simulink model "a1_climbing"  (R2022b)
settings: Solver=VariableStepAuto  StartTime=0.0  StopTime=5  RelTol=1e-3
values from neighbouring files (symbols this model uses):
  m = 12    [MPC_Controller.m]    (also in QP_Controller.m; TASK1_rotating_mpc.m; TASK1_walking_backward_mpc.m; TASK1_walking_forward_mpc.m)
  N = 10    [MPC_Controller.m]
undefined symbols (not defined in the file or in its folder): climbing_mpc, X, Y, Z
libraries: sm_lib x206, nesl_utility x122, simulink x1
(part 6 of 6)

== system a1_climbing/Stand Controller/Subsystem9 ==
  angle : Inport
  velocity : Inport  Port=2
  Add : Sum
  Constant1 : Constant  Value=-0.5
  Constant2 : Constant  Value=-5
  Constant3 : Constant  Value=0
  Product : Product
  Product1 : Product
  Saturation : Saturate  UpperLimit=33.5  LowerLimit=-33.5
  Subtract : Sum  Inputs=+-
  Torque : Outport
  wires:
  angle/1 -> Subtract/1
  Constant2/1 -> Product/2
  Subtract/1 -> Product/1
  Constant1/1 -> Product1/2
  velocity/1 -> Product1/1
  Product1/1 -> Add/2
  Product/1 -> Add/1
  Constant3/1 -> Subtract/2
  Add/1 -> Saturation/1
  Saturation/1 -> Torque/1

== system a1_climbing/Walk Controller/Convert Forces to Torque1 ==
  F : Inport
  RR_Ang_Vec : Inport  Port=2
  RL_Ang_Vec : Inport  Port=3
  FL_Ang_Vec : Inport  Port=4
  FR_Ang_Vec : Inport  Port=5
  Force to Torque : MATLAB Function  TreatAsAtomicUnit=on
  Tau_FL : Outport
  Tau_RL : Outport  Port=2
  Tau_FR : Outport  Port=3
  Tau_RR : Outport  Port=4
  wires:
  F/1 -> Force to Torque/1(F)
  Force to Torque/1(Tau_RR) -> Tau_RR/1
  Force to Torque/2(Tau_FR) -> Tau_FR/1
  Force to Torque/3(Tau_FL) -> Tau_FL/1
  Force to Torque/4(Tau_RL) -> Tau_RL/1
  RR_Ang_Vec/1 -> Force to Torque/2(RR_ang_vec)
  RL_Ang_Vec/1 -> Force to Torque/3(RL_ang_vec)
  FL_Ang_Vec/1 -> Force to Torque/4(FL_ang_vec)
  FR_Ang_Vec/1 -> Force to Torque/5(FR_ang_vec)

== system a1_climbing/Walk Controller/Rigid Body Controller ==
  FL Pos : Inport
  RL Pos : Inport  Port=2
  FR Pos : Inport  Port=3
  RR Pos : Inport  Port=4
  COM_pos : Inport  Port=5
  COM_vel : Inport  Port=6
  COM_ang_vel : Inport  Port=7
  Rot : Inport  Port=8
  v_desired : Inport  Port=9
  T_stance : Inport  Port=10
  Clock : Clock
  Interpreted MATLAB Function : MATLABFcn  MATLABFcn=climbing_mpc(u)  OutputDimensions=12  Output1D=off
  Memory : Memory
  Mux : Mux  Inputs=11
  Rotation Matrix to Eul : MATLAB Function  TreatAsAtomicUnit=on
  Scope : Scope  NumInputPorts=5
  Selector : Selector  InputPortWidth=12  IndexOptions=Index vector (dialog)  Indices=[1 3]  OutputSizes=1
  Zero-Order Hold : ZeroOrderHold  SampleTime=.05
  u : Outport
  wires:
  COM_pos/1 -> Mux/1
  COM_vel/1 -> Mux/2
  COM_ang_vel/1 -> Mux/4
  FL Pos/1 -> Mux/5
  RL Pos/1 -> Mux/6
  FR Pos/1 -> Mux/7
  RR Pos/1 -> Mux/8
  Rot/1 -> Rotation Matrix to Eul/1(u)
  Rotation Matrix to Eul/1(y) -> Mux/3
  Interpreted MATLAB Function/1 -> Memory/1
  Memory/1 -> Selector/1, u/1
  Mux/1 -> Zero-Order Hold/1
  Zero-Order Hold/1 -> Interpreted MATLAB Function/1
  Clock/1 -> Mux/9
  Selector/1 -> Scope/1
  v_desired/1 -> Mux/10
  T_stance/1 -> Mux/11

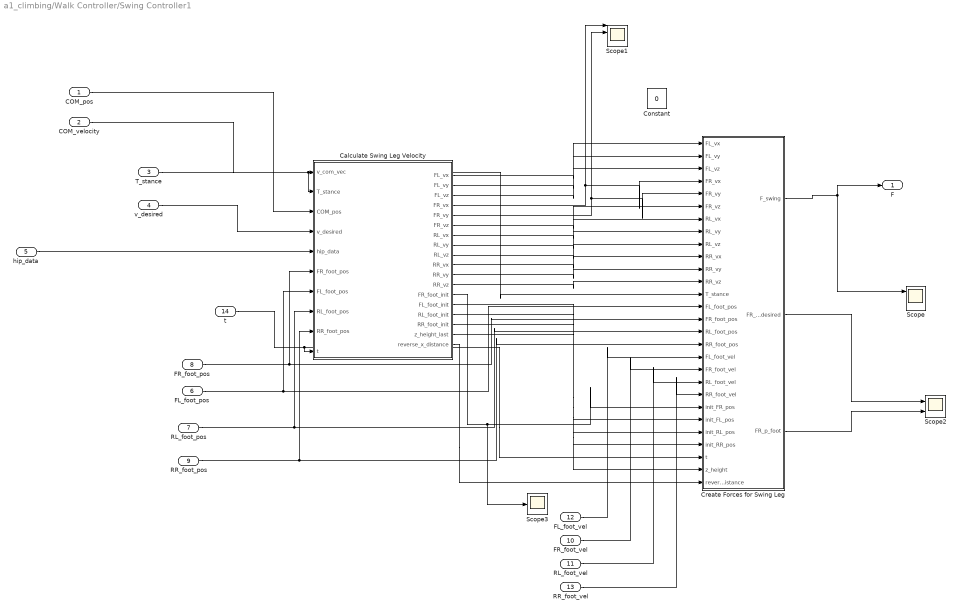
== system a1_climbing/Walk Controller/Swing Controller1 ==
  COM_pos : Inport
  COM_velocity : Inport  Port=2
  T_stance : Inport  Port=3
  v_desired : Inport  Port=4
  hip_data : Inport  Port=5
  FL_foot_pos : Inport  Port=6
  RL_foot_pos : Inport  Port=7
  FR_foot_pos : Inport  Port=8
  RR_foot_pos : Inport  Port=9
  FR_foot_vel : Inport  Port=10
  RL_foot_vel : Inport  Port=11
  FL_foot_vel : Inport  Port=12
  RR_foot_vel : Inport  Port=13
  t : Inport  Port=14
  Calculate Swing Leg Velocity : MATLAB Function  TreatAsAtomicUnit=on  SystemSampleTime=0.2
  Constant : Constant  Value=0
  Create Forces for Swing Leg : MATLAB Function  TreatAsAtomicUnit=on
  Scope : Scope  NumInputPorts=3
  Scope1 : Scope  NumInputPorts=4
  Scope2 : Scope  NumInputPorts=2
  Scope3 : Scope
  F : Outport
  wires:
  T_stance/1 -> Calculate Swing Leg Velocity/2(T_stance), Create Forces for Swing Leg/13(T_stance)
  v_desired/1 -> Calculate Swing Leg Velocity/4(v_desired)
  Create Forces for Swing Leg/1(F_swing) -> Scope/1, F/1
  t/1 -> Calculate Swing Leg Velocity/10(t), Create Forces for Swing Leg/26(t)
  hip_data/1 -> Calculate Swing Leg Velocity/5(hip_data)
  Calculate Swing Leg Velocity/12(RR_vz) -> Create Forces for Swing Leg/12(RR_vz)
  Calculate Swing Leg Velocity/11(RR_vy) -> Create Forces for Swing Leg/11(RR_vy)
  Calculate Swing Leg Velocity/10(RR_vx) -> Create Forces for Swing Leg/10(RR_vx)
  Calculate Swing Leg Velocity/9(RL_vz) -> Create Forces for Swing Leg/9(RL_vz)
  Calculate Swing Leg Velocity/8(RL_vy) -> Create Forces for Swing Leg/8(RL_vy)
  Calculate Swing Leg Velocity/7(RL_vx) -> Create Forces for Swing Leg/7(RL_vx)
  Calculate Swing Leg Velocity/6(FR_vz) -> Create Forces for Swing Leg/6(FR_vz)
  Calculate Swing Leg Velocity/5(FR_vy) -> Create Forces for Swing Leg/5(FR_vy), Scope1/2
  Calculate Swing Leg Velocity/4(FR_vx) -> Create Forces for Swing Leg/4(FR_vx), Scope1/1
  Calculate Swing Leg Velocity/3(FL_vz) -> Create Forces for Swing Leg/3(FL_vz)
  Calculate Swing Leg Velocity/2(FL_vy) -> Create Forces for Swing Leg/2(FL_vy)
  Calculate Swing Leg Velocity/1(FL_vx) -> Create Forces for Swing Leg/1(FL_vx)
  FR_foot_pos/1 -> Create Forces for Swing Leg/15(FR_foot_pos), Calculate Swing Leg Velocity/6(FR_foot_pos)
  RL_foot_pos/1 -> Calculate Swing Leg Velocity/8(RL_foot_pos), Create Forces for Swing Leg/16(RL_foot_pos)
  RR_foot_pos/1 -> Create Forces for Swing Leg/17(RR_foot_pos), Calculate Swing Leg Velocity/9(RR_foot_pos)
  FL_foot_vel/1 -> Create Forces for Swing Leg/18(FL_foot_vel)
  FR_foot_vel/1 -> Create Forces for Swing Leg/19(FR_foot_vel)
  RL_foot_vel/1 -> Create Forces for Swing Leg/20(RL_foot_vel)
  RR_foot_vel/1 -> Create Forces for Swing Leg/21(RR_foot_vel)
  Create Forces for Swing Leg/2(FR_p_desired) -> Scope2/1
  COM_velocity/1 -> Calculate Swing Leg Velocity/1(v_com_vec)
  Calculate Swing Leg Velocity/13(FR_foot_init) -> Scope3/1, Create Forces for Swing Leg/22(init_FR_pos)
  Create Forces for Swing Leg/3(FR_p_foot) -> Scope2/2
  FL_foot_pos/1 -> Calculate Swing Leg Velocity/7(FL_foot_pos), Create Forces for Swing Leg/14(FL_foot_pos)
  Calculate Swing Leg Velocity/14(FL_foot_init) -> Create Forces for Swing Leg/23(init_FL_pos)
  Calculate Swing Leg Velocity/15(RL_foot_init) -> Create Forces for Swing Leg/24(init_RL_pos)
  Calculate Swing Leg Velocity/16(RR_foot_init) -> Create Forces for Swing Leg/25(init_RR_pos)
  COM_pos/1 -> Calculate Swing Leg Velocity/3(COM_pos)
  Calculate Swing Leg Velocity/17(z_height_last) -> Create Forces for Swing Leg/27(z_height)
  Calculate Swing Leg Velocity/18(reverse_x_distance) -> Create Forces for Swing Leg/28(reverse_x_distance)

== matlab function a1_climbing/Rear Right Leg/Separate Torques ==
  data: torque_vector input; hip_torque output; thigh_torque output; calf_torque output
function [hip_torque, thigh_torque, calf_torque] = fcn(torque_vector)

hip_torque = torque_vector(1);
thigh_torque = torque_vector(2);
calf_torque = torque_vector(3);

== matlab function a1_climbing/Front Left Leg/Separate Torques ==
  data: torque_vector input; hip_torque output; thigh_torque output; calf_torque output
function [hip_torque, thigh_torque, calf_torque] = fcn(torque_vector)

hip_torque = torque_vector(1);
thigh_torque = torque_vector(2);
calf_torque = torque_vector(3);

== matlab function a1_climbing/Stand Controller/MATLAB Function ==
  data: angle_vector input; hip_angle output; thigh_angle output; calf_angle output
function [hip_angle, thigh_angle, calf_angle] = fcn(angle_vector)

hip_angle = angle_vector(1);
thigh_angle = angle_vector(2);
calf_angle = angle_vector(3);

== matlab function a1_climbing/Stand Controller/MATLAB Function1 ==
  data: velocity_vector input; hip_velocity output; thigh_velocity output; calf_velocity output
function [hip_velocity, thigh_velocity, calf_velocity] = fcn(velocity_vector)

hip_velocity = velocity_vector(1);
thigh_velocity = velocity_vector(2);
calf_velocity = velocity_vector(3);

== matlab function a1_climbing/Stand Controller/MATLAB Function2 ==
  data: angle_vector input; hip_angle output; thigh_angle output; calf_angle output
function [hip_angle, thigh_angle, calf_angle] = fcn(angle_vector)

hip_angle = angle_vector(1);
thigh_angle = angle_vector(2);
calf_angle = angle_vector(3);

== matlab function a1_climbing/Stand Controller/MATLAB Function3 ==
  data: velocity_vector input; hip_velocity output; thigh_velocity output; calf_velocity output
function [hip_velocity, thigh_velocity, calf_velocity] = fcn(velocity_vector)

hip_velocity = velocity_vector(1);
thigh_velocity = velocity_vector(2);
calf_velocity = velocity_vector(3);

== matlab function a1_climbing/Stand Controller/MATLAB Function4 ==
  data: angle_vector input; hip_angle output; thigh_angle output; calf_angle output
function [hip_angle, thigh_angle, calf_angle] = fcn(angle_vector)

hip_angle = angle_vector(1);
thigh_angle = angle_vector(2);
calf_angle = angle_vector(3);

== matlab function a1_climbing/Stand Controller/MATLAB Function5 ==
  data: velocity_vector input; hip_velocity output; thigh_velocity output; calf_velocity output
function [hip_velocity, thigh_velocity, calf_velocity] = fcn(velocity_vector)

hip_velocity = velocity_vector(1);
thigh_velocity = velocity_vector(2);
calf_velocity = velocity_vector(3);

== matlab function a1_climbing/Stand Controller/MATLAB Function6 ==
  data: angle_vector input; hip_angle output; thigh_angle output; calf_angle output
function [hip_angle, thigh_angle, calf_angle] = fcn(angle_vector)

hip_angle = angle_vector(1);
thigh_angle = angle_vector(2);
calf_angle = angle_vector(3);

== matlab function a1_climbing/Stand Controller/MATLAB Function7 ==
  data: velocity_vector input; hip_velocity output; thigh_velocity output; calf_velocity output
function [hip_velocity, thigh_velocity, calf_velocity] = fcn(velocity_vector)

hip_velocity = velocity_vector(1);
thigh_velocity = velocity_vector(2);
calf_velocity = velocity_vector(3);

== matlab function a1_climbing/Walk Controller/Combine Forces ==
  data: t input; T_stance input; F output; rigid_body_forces input; swing_forces input
function F = fcn(t, T_stance, rigid_body_forces, swing_forces)
%#codegen
intervals = 0:T_stance:10;

interval_idx = discretize(t, intervals);

if mod(interval_idx(1), 2) == 0
    F = [rigid_body_forces(1:3); -swing_forces(4:6); -swing_forces(7:9); rigid_body_forces(10:12)];
else
    F = [-swing_forces(1:3); rigid_body_forces(4:6); rigid_body_forces(7:9); -swing_forces(10:12)];
end

== matlab function a1_climbing/Walk Controller/Rigid Body Controller/Rotation Matrix to Eul ==
  data: u input; y output
function y = fcn(u)
y = rotm2eul(u);

== matlab function a1_climbing/Walk Controller/Swing Controller1/Calculate Swing Leg Velocity ==
  data: FL_vx output; FL_vy output; v_com_vec input; FL_vz output; T_stance input; COM_pos input; v_desired input; hip_data input; FR_foot_pos input; FL_foot_pos input; RL_foot_pos input; FR_vx output; FR_vy output; FR_vz output; RL_vx output; RL_vy output; RL_vz output; RR_vx output; RR_vy output; RR_vz output; FR_foot_init output; RR_foot_pos input; FL_foot_init output; RL_foot_init output; RR_foot_init output; t input; z_height_last output; reverse_x_distance output
function [FL_vx,FL_vy,FL_vz,FR_vx,FR_vy,FR_vz,RL_vx,RL_vy,RL_vz,RR_vx,RR_vy,RR_vz,FR_foot_init,FL_foot_init,RL_foot_init,RR_foot_init,z_height_last,reverse_x_distance] = fcn(v_com_vec,T_stance,COM_pos,v_desired,hip_data,FR_foot_pos,FL_foot_pos,RL_foot_pos,RR_foot_pos,t)

z_height = 0.14; 
z_height_last = z_height;

FL_hip_pos = hip_data(1:3);
FR_hip_pos = hip_data(4:6);
RL_hip_pos = hip_data(7:9);
RR_hip_pos = hip_data(10:12);
FR_foot_init = FR_foot_pos;
FL_foot_init = FL_foot_pos;
RL_foot_init = RL_foot_pos;
RR_foot_init = RR_foot_pos;
reverse_x_distance = 0.03; 

% Find K_step - this value can be tuned with z_com_desired
z_com_desired = 0.3;
g = 9.81;
K_step = sqrt(z_com_desired/g);

%% FL
% Find P_foot_desired - FL
FL_hip_pos(3) = 0;
FL_p_foot_desired_end = FL_hip_pos+(T_stance/2)*v_desired+K_step*(v_com_vec-v_desired);
FL_p_foot_desired_end(2) = FL_p_foot_desired_end(2)+0.06;
FL_foot_pos(1) = FL_foot_pos(1)-2*reverse_x_distance;

if FL_p_foot_desired_end(1) > 0.41
    FL_p_foot_desired_end(3) = 0.1;
    half_step = (FL_p_foot_desired_end - FL_foot_pos)/2+[0;0;z_height];
elseif FL_p_foot_desired_end(1) > 0.61
    FL_p_foot_desired_end(3) = 0.2;
    half_step = (FL_p_foot_desired_end - FL_foot_pos)/2+[0;0;z_height];
else
   FL_p_foot_desired_end(3) = 0;
   half_step = (FL_p_foot_desired_end - FL_foot_pos)/2+[0;0;z_height];
end

% Create Trajectory 
half_step_time = T_stance/2;
v = half_step/half_step_time;

FL_vx = v(1);
FL_vy = v(2);
FL_vz = v(3);

%% FR
% Find P_foot_desired - FR
FR_hip_pos(3) = 0;
FR_p_foot_desired_end = FR_hip_pos+(T_stance/2)*v_desired+K_step*(v_com_vec-v_desired);
FR_p_foot_desired_end(2) = FR_p_foot_desired_end(2)-0.06;
FR_foot_pos(1) = FR_foot_pos(1)-2*reverse_x_distance;
if FR_p_foot_desired_end(1) > 0.41
    FR_p_foot_desired_end(3) = 0.1;
    half_step = (FR_p_foot_desired_end - FR_foot_pos)/2+[0;0;z_height];
elseif FR_p_foot_desired_end(1) > 0.61
    FR_p_foot_desired_end(3) = 0.2;
    half_step = (FR_p_foot_desired_end - FR_foot_pos)/2+[0;0;z_height];
else
   FR_p_foot_desired_end(3) = 0;
   half_step = (FR_p_foot_desired_end - FR_foot_pos)/2+[0;0;z_height];
end


% Create Trajectory 
half_step_time = T_stance/2;
v = half_step/half_step_time;

FR_vx = v(1);
FR_vy = v(2);
FR_vz = v(3);

%% RL
% Find P_foot_desired - RL
RL_hip_pos(3) = 0;
RL_p_foot_desired_end = RL_hip_pos+(T_stance/2)*v_desired+K_step*(v_com_vec-v_desired);
RL_p_foot_desired_end(2) = RL_p_foot_desired_end(2)+0.06;
RL_p_foot_desired_end(3) = 0;
RL_foot_pos(1) = RL_foot_pos(1)-2*reverse_x_distance;
if RL_p_foot_desired_end(1) > 0.41
    RL_p_foot_desired_end(3) = 0.1;
    half_step = (RL_p_foot_desired_end - RL_foot_pos)/2+[0;0;z_height];
elseif RL_p_foot_desired_end(1) > 0.61
    RL_p_foot_desired_end(3) = 0.2;
    half_step = (RL_p_foot_desired_end - RL_foot_pos)/2+[0;0;z_height];
else
   RL_p_foot_desired_end(3) = 0;
   half_step = (RL_p_foot_desired_end - RL_foot_pos)/2+[0;0;z_height];
end

% Create Trajectory 
half_step_time = T_stance/2;
v = half_step/half_step_time;

RL_vx = v(1);
RL_vy = v(2);
RL_vz = v(3);


%% RR
% Find P_foot_desired - RR
RR_hip_pos(3) = 0;
RR_p_foot_desired_end = RR_hip_pos+(T_stance/2)*v_desired+K_step*(v_com_vec-v_desired);
RR_p_foot_desired_end(2) = RR_p_foot_desired_end(2)-0.06;
RR_foot_pos(1) = RR_foot_pos(1)-2*reverse_x_distance;
RR_p_foot_desired_end(3) = 0;

% Create Trajectory 
if RR_p_foot_desired_end(1) > 0.41
    RR_p_foot_desired_end(3) = 0.1;
    half_step = (RR_p_foot_desired_end - RR_foot_pos)/2+[0;0;z_height];
elseif RR_p_foot_desired_end(1) > 0.61
    RR_p_foot_desired_end(3) = 0.2;
    half_step = (RR_p_foot_desired_end - RR_foot_pos)/2+[0;0;z_height];
else
   RR_p_foot_desired_end(3) = 0;
   half_step = (RR_p_foot_desired_end - RR_foot_pos)/2+[0;0;z_height];
end

half_step_time = T_stance/2;
v = half_step/half_step_time;

RR_vx = v(1);
RR_vy = v(2);
RR_vz = v(3);

== matlab function a1_climbing/Walk Controller/Swing Controller1/Create Forces for Swing Leg ==
  data: FL_vx input; F_swing output; FL_vy input; FL_vz input; FR_vx input; FR_vy input; FR_vz input; RL_vx input; RL_vy input; RL_vz input; RR_vx input; RR_vy input; RR_vz input; T_stance input; FL_foot_pos input; FR_foot_pos input; RL_foot_pos input; RR_foot_pos input; FL_foot_vel input; FR_foot_vel input; RL_foot_vel input; RR_foot_vel input; init_FR_pos input; init_FL_pos input; init_RL_pos input; init_RR_pos input; t input; FR_p_desired output; FR_p_foot output; z_height input; reverse_x_distance input
function [F_swing,FR_p_desired,FR_p_foot]  = fcn(FL_vx,FL_vy,FL_vz,FR_vx,FR_vy,FR_vz,RL_vx,RL_vy,RL_vz,RR_vx,RR_vy,RR_vz,T_stance,FL_foot_pos,FR_foot_pos,RL_foot_pos,RR_foot_pos,FL_foot_vel,FR_foot_vel,RL_foot_vel,RR_foot_vel,init_FR_pos,init_FL_pos,init_RL_pos,init_RR_pos,t,z_height, reverse_x_distance)

% These are the desired velocity values calculated from the previous block
% These are the desired velocity for each foot position through the swing
FL_v_desired = [FL_vx;FL_vy;FL_vz];
FR_v_desired = [FR_vx;FR_vy;FR_vz];
RL_v_desired = [RL_vx;RL_vy;RL_vz];
RR_v_desired = [RR_vx;RR_vy;RR_vz];

% These are the actual current foot position and velocity - these update
% continously
FL_p_foot = FL_foot_pos(1:3);
FL_v_foot = FL_foot_vel(1:3);
FR_p_foot = FR_foot_pos(1:3);
FR_v_foot = FR_foot_vel(1:3);
RL_p_foot = RL_foot_pos(1:3);
RL_v_foot = RL_foot_vel(1:3);
RR_p_foot = RR_foot_pos(1:3);
RR_v_foot = RR_foot_vel(1:3);

steps = 0:T_stance:10; 

if t <= 0.2 
    FL_px = 0;
    FL_py = 0; 
    FL_pz = 0;
    FR_px = 0;
    FR_py = 0; 
    FR_pz = 0; 
    RL_px = 0;
    RL_py = 0; 
    RL_pz = 0; 
    RR_px = 0;
    RR_py = 0; 
    RR_pz = 0; 
    
else
    step_index = discretize(t,steps);
    delta_t = t-steps(step_index);
   
    % Find the DELTA desired position of the foot using the time
    % This wil be added to the intitial foot position
    % Note that the delta_x will be negative until we hit the reverse x
    % distance
    FL_py = FL_vy*delta_t; 
    FL_pz = FL_vz*delta_t;
    FR_py = FR_vy*delta_t; 
    FR_pz = FR_vz*delta_t; 
    RL_py = RL_vy*delta_t; 
    RL_pz = RL_vz*delta_t; 
    RR_py = RR_vy*delta_t; 
    RR_pz = RR_vz*delta_t; 

    FL_T_back = abs(reverse_x_distance/FL_vx);
    FR_T_back = abs(reverse_x_distance/FR_vx);
    RL_T_back = abs(reverse_x_distance/RL_vx);
    RR_T_back = abs(reverse_x_distance/RR_vx);

    % Reverse direction when you reverse_x_distance
    if delta_t > FL_T_back
        FL_px = -reverse_x_distance+FL_vx*(delta_t-FL_T_back);
        FL_v_desired(1) = FL_v_desired(1); % Set velocity  to positive
    else
        FL_px = -FL_vx*delta_t;
        FL_v_desired(1) = -FL_v_desired(1);
    end

    if delta_t > FR_T_back
        FR_px = -reverse_x_distance+FR_vx*(delta_t-FR_T_back);
        FR_v_desired(1) = FR_v_desired(1); % Set velocity  to positive
    else
        FR_px = -FR_vx*delta_t;
        FR_v_desired(1) = -FR_v_desired(1);
    end


    if delta_t > RL_T_back
        RL_px = -reverse_x_distance+RL_vx*(delta_t-RL_T_back);
        RL_v_desired(1) = RL_v_desired(1); % Set velocity  to positive
    else
        RL_px = -RL_vx*delta_t;
        RL_v_desired(1) = -RL_v_desired(1);
    end

    if delta_t > RR_T_back
        RR_px = -reverse_x_distance+RR_vx*(delta_t-RR_T_back);
        RR_v_desired(1) = RR_v_desired(1); % Set velocity  to positive
    else
        RR_px = -RR_vx*delta_t;
        RR_v_desired(1) = -RR_v_desired(1);
    end

    % Reverse direction when you hit z_height
    if FL_pz > z_height
        FL_pz = z_height-FL_vz*(delta_t-T_stance/2);
        FL_v_desired(3) = -FL_v_desired(3);
    end
    if FR_pz > z_height
        FR_pz = z_height-FR_vz*(delta_t-T_stance/2);
        FR_v_desired(3) = -FR_v_desired(3);
    end
    if RL_pz > z_height
        RL_pz = z_height-RL_vz*(delta_t-T_stance/2);
        RL_v_desired(3) = -RL_v_desired(3);
    end
    if RR_pz > z_height
        RR_pz = z_height-RR_vz*(delta_t-T_stance/2);
        RR_v_desired(3) = -RR_v_desired(3);
    end




end

z_offset = 0.01;
% Foot pos desired at time t 
FL_p_desired = [init_FL_pos(1); init_FL_pos(2); init_FL_pos(3)] + [FL_px;FL_py;FL_pz];
FR_p_desired = [init_FR_pos(1); init_FR_pos(2); init_FR_pos(3)] + [FR_px;FR_py;FR_pz];
RL_p_desired = [init_RL_pos(1); init_RL_pos(2); init_RL_pos(3)] + [RL_px;RL_py;RL_pz];
RR_p_desired = [init_RR_pos(1); init_RR_pos(2); init_RR_pos(3)] + [RR_px;RR_py;RR_pz];

FL_p_foot = FL_p_foot - [0;0;z_offset];
FR_p_foot = FR_p_foot - [0;0;z_offset];
RL_p_foot = RL_p_foot - [0;0;z_offset];
RR_p_foot = RR_p_foot - [0;0;z_offset];

% Find the force using a PD controller - FL
KP = [400;400;400]; 
KD = [10;10;10]; 
F_swing_FL = KP.*(FL_p_desired-FL_p_foot)+KD.*(FL_v_desired-FL_v_foot);
F_swing_FR = KP.*(FR_p_desired-FR_p_foot)+KD.*(FR_v_desired-FR_v_foot);
F_swing_RL = KP.*(RL_p_desired-RL_p_foot)+KD.*(RL_v_desired-RL_v_foot);
F_swing_RR = KP.*(RR_p_desired-RR_p_foot)+KD.*(RR_v_desired-RR_v_foot);

F_swing = [F_swing_FL;F_swing_RL; F_swing_FR; F_swing_RR];

== matlab function a1_climbing/Walk Controller/MATLAB Function ==
  data: P input; pos_d output; v_d input
function pos_d = fcn(P,v_d)
dt = 0.05;
pos_d = P(1)+ 10*dt*v_d(1);

== matlab function a1_climbing/MATLAB Function ==
  data: t input; FL output; torques_stand input; torques_walk input; RL output; FR output; RR output
function [FL, RL, FR, RR] = fcn(t, torques_stand, torques_walk)
%#codegen
if t < 1
    FL = torques_stand(1:3);
    RL = torques_stand(4:6);
    FR = torques_stand(7:9);
    RR = torques_stand(10:12);
else
    FL = torques_walk(1:3);
    RL = torques_walk(4:6);
    FR = torques_walk(7:9);
    RR = torques_walk(10:12);
end

== matlab function a1_climbing/Walk Controller/Convert Forces to Torque1/Force to Torque ==
  data: F input; Tau_RR output; RR_ang_vec input; RL_ang_vec input; FL_ang_vec input; FR_ang_vec input; Tau_FR output; Tau_FL output; Tau_RL output
function [Tau_RR,Tau_FR,Tau_FL,Tau_RL]= fcn(F,RR_ang_vec,RL_ang_vec,FL_ang_vec,FR_ang_vec)
    % TODO - Convert forces to torques using the inverse jacobian
    % Get forces from the force vector 
    % NOTE - VERIFY THAT THESE ARE THE CORRECT VECTORS (I am unsure)
    F_FL = F(1:3);
    F_RL = F(4:6);
    F_FR = F(7:9);
    F_RR = F(10:12);

    l1=0.045; % hip length
    l2=0.2; % thigh length
    l3=0.2; % calf length
    

    %% Calculate the force for the RR leg - NOTE: The right legs have the
    % same jacobians
    q = RR_ang_vec; %
    leg = 4;
  
    if leg==1 || leg==3 % left leg has sideSign 1
        sideSign=1;
    else
        sideSign=-1; % right leg has sideSign -1
    end
    s1=sin(q(1)); % for hip joint
    s2=sin(q(2)); % for thigh joint
    s3=sin(q(3)); % for calf joint

    c1=cos(q(1)); % for hip joint
    c2=cos(q(2)); % for thigh joint
    c3=cos(q(3)); % for calf joint
    
    c23=c2*c3-s2*s3;
    s23=s2*c3+c2*s3;
    J = eye(3);
    J(1,1)=0;
    J(2,1)=-sideSign*l1*s1+l2*c2*c1+l3*c23*c1;
    J(3,1)=sideSign*l1*c1+l2*c2*s1+l3*c23*s1;
    
    J(1,2)=-l3*c23-l2*c2;
    J(2,2)=-l2*s2*s1-l3*s23*s1;
    J(3,2)=l2*s2*c1+l3*s23*c1;

    J(1,3)=-l3*c23;
    J(2,3)=-l3*s23*s1;
    J(3,3)=l3*s23*c1;
    
    inJ_R_RR = transpose(J);
    Tau_RR = -inJ_R_RR*F_RR;

  
    %% Calculate the force for the FR leg - NOTE: The right legs have the
    % same jacobians
    q = FR_ang_vec; %
    leg = 2;
  
    if leg==1 || leg==3 % left leg has sideSign 1
        sideSign=1;
    else
        sideSign=-1; % right leg has sideSign -1
    end
    s1=sin(q(1)); % for hip joint
    s2=sin(q(2)); % for thigh joint
    s3=sin(q(3)); % for calf joint

    c1=cos(q(1)); % for hip joint
    c2=cos(q(2)); % for thigh joint
    c3=cos(q(3)); % for calf joint
    
    c23=c2*c3-s2*s3;
    s23=s2*c3+c2*s3;

    J(1,1)=0;
    J(2,1)=-sideSign*l1*s1+l2*c2*c1+l3*c23*c1;
    J(3,1)=sideSign*l1*c1+l2*c2*s1+l3*c23*s1;
    
    J(1,2)=-l3*c23-l2*c2;
    J(2,2)=-l2*s2*s1-l3*s23*s1;
    J(3,2)=l2*s2*c1+l3*s23*c1;

    J(1,3)=-l3*c23;
    J(2,3)=-l3*s23*s1;
    J(3,3)=l3*s23*c1;

    inJ_R_FR = transpose(J);
    Tau_FR = -inJ_R_FR*F_FR;

    %% Calculate the force for the FL leg - NOTE: The right legs have the
    % same jacobians
    q = FL_ang_vec; %
    leg = 1;
  
    if leg==1 || leg==3 % left leg has sideSign 1
        sideSign=1;
    else
        sideSign=-1; % right leg has sideSign -1
    end
    s1=sin(q(1)); % for hip joint
    s2=sin(q(2)); % for thigh joint
    s3=sin(q(3)); % for calf joint

    c1=cos(q(1)); % for hip joint
    c2=cos(q(2)); % for thigh joint
    c3=cos(q(3)); % for calf joint
    
    c23=c2*c3-s2*s3;
    s23=s2*c3+c2*s3;

    J(1,1)=0;
    J(2,1)=-sideSign*l1*s1+l2*c2*c1+l3*c23*c1;
    J(3,1)=sideSign*l1*c1+l2*c2*s1+l3*c23*s1;
    
    J(1,2)=-l3*c23-l2*c2;
    J(2,2)=-l2*s2*s1-l3*s23*s1;
    J(3,2)=l2*s2*c1+l3*s23*c1;

    J(1,3)=-l3*c23;
    J(2,3)=-l3*s23*s1;
    J(3,3)=l3*s23*c1;

    inJ_R_FL = transpose(J);
    Tau_FL = -inJ_R_FL*F_FL;


    %% Calculate the force for the RL leg - NOTE: The right legs have the
    % same jacobians
    q = RL_ang_vec; %
    leg = 3;
  
    if leg==1 || leg==3 % left leg has sideSign 1
        sideSign=1;
    else
        sideSign=-1; % right leg has sideSign -1
    end
    s1=sin(q(1)); % for hip joint
    s2=sin(q(2)); % for thigh joint
    s3=sin(q(3)); % for calf joint

    c1=cos(q(1)); % for hip joint
    c2=cos(q(2)); % for thigh joint
    c3=cos(q(3)); % for calf joint
    
    c23=c2*c3-s2*s3;
    s23=s2*c3+c2*s3;

    J(1,1)=0;
    J(2,1)=-sideSign*l1*s1+l2*c2*c1+l3*c23*c1;
    J(3,1)=sideSign*l1*c1+l2*c2*s1+l3*c23*s1;
    
    J(1,2)=-l3*c23-l2*c2;
    J(2,2)=-l2*s2*s1-l3*s23*s1;
    J(3,2)=l2*s2*c1+l3*s23*c1;

    J(1,3)=-l3*c23;
    J(2,3)=-l3*s23*s1;
    J(3,3)=l3*s23*c1;

    inJ_R_RL = transpose(J);
    Tau_RL = -inJ_R_RL*F_RL;

== matlab function a1_climbing/Rear Left Leg/Separate Torques ==
  data: torque_vector input; hip_torque output; thigh_torque output; calf_torque output
function [hip_torque, thigh_torque, calf_torque] = fcn(torque_vector)

hip_torque = torque_vector(1);
thigh_torque = torque_vector(2);
calf_torque = torque_vector(3);

== matlab function a1_climbing/Front Right Leg/Separate Torques ==
  data: torque_vector input; hip_torque output; thigh_torque output; calf_torque output
function [hip_torque, thigh_torque, calf_torque] = fcn(torque_vector)

hip_torque = torque_vector(1);
thigh_torque = torque_vector(2);
calf_torque = torque_vector(3);
